simulink model "sfcndemo_csparam"  (Simulink 7.6)
settings: Solver=FixedStepDiscrete  StartTime=0.0  StopTime=Inf  RelTol=1e-3
PostLoadFcn:
  | K1 = 2; K2 = int8(3); MYTYPE = Simulink.AliasType('single');
Description:
  | Context-Sensitive Parameters in C-MEX S-functions
settings Model: Creator=The MathWorks Inc.  CovMetricSettings=d  ExtModeAutoUpdateStatusClock=off  TunableVars=K1,K2  TunableVarsStorageClass=ExportedGlobal,ExportedGlobal  TunableVarsTypeQualifier=,
settings DataIOCC: SaveOutput=off  SaveTime=off  SignalLoggingName=sigsOut
settings OptimizationCC: InlineParams=on  StateBitsets=on  DataBitsets=on  UseTempVars=on  InitFltsAndDblsToZero=on  BufferReusableBoundary=off
settings DebuggingCC: SaveWithParameterizedLinksMsg=none  CheckExecutionContextPreStartOutputMsg=on  CheckExecutionContextRuntimeOutputMsg=on  SolverPrmCheckMsg=none  MultiTaskDSMMsg=warning  MultiTaskCondExecSysMsg=none
settings SFSimCC: SimParseCustomCode=off
settings RTWCC: TLCOptions=-p0  GenerateReport=on  ProcessScript=grt_make_rtw_hook  LaunchReport=on  IncludeERTFirstTime=on
settings CodeAppCC: ForceParamTrailComments=on  CustomSymbolStrFcn=$F$N$M
settings GRTTargetCC: TargetFcnLib=ansi_tfl_tmw.mat

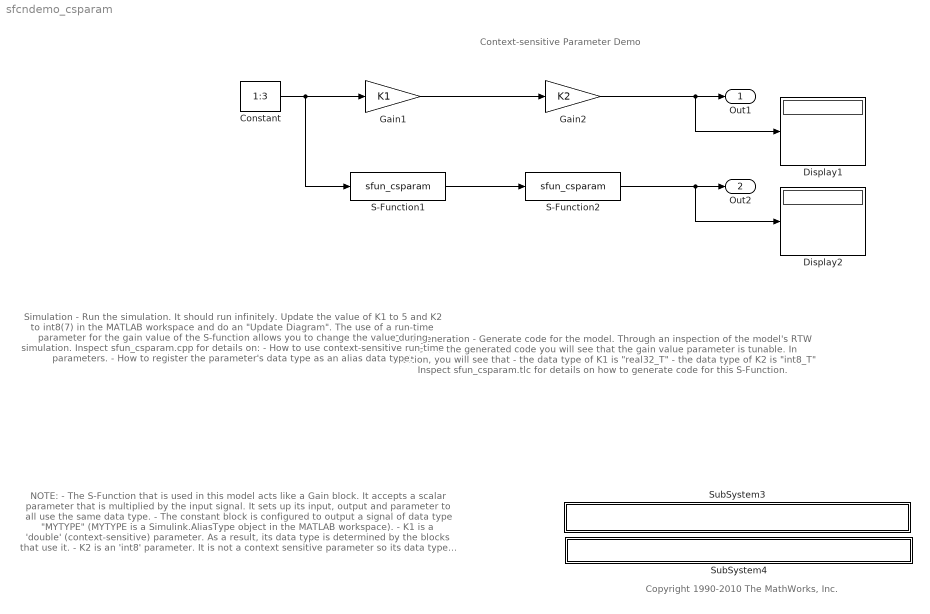
== system sfcndemo_csparam ==
  note: Code generation -
      | Generate code for the model. Through an inspection of the
      | model's RTW file and the generated code you will see that the
      | gain value parameter is tunable.  In addition, you will see that
      | - the data type of K1 is "real32_T"
      | - the data type of K2 is "int8_T"
      |
      | Inspect sfun_csparam.tlc for details on how to generate code
      | for this S-Function.
  note: Simulation -
      | Run the simulation. It should run infinitely.
      | Update the value of K1 to 5 and K2 to int8(7)
      | in the MATLAB workspace and do an "Update Diagram".
      | The use of a run-time parameter for the gain value of the
      | S-function allows you to change the value during simulation.
      |
      | Inspect sfun_csparam.cpp for details on:
      | - How to use context-sensitive run-time parameters.
      | - How to register the parameter's data type as an alias data type.
  note: Context-sensitive Parameter Demo
  note: NOTE:
      | - The S-Function that is used in this model acts like a Gain block.
      |    It accepts a scalar parameter that is multiplied by the input signal.
      |    It sets up its input, output and parameter to all use the same data type.
      | - The constant block is configured to output a signal of data type "MYTYPE"
      |    (MYTYPE is a Simulink.AliasType object in the MATLAB workspace).
      | - K1 is a 'double' (context-sensitive) parameter.
      |    As a result, its data type is determined by the blocks that use it.
      | - K2 is an 'int8' parameter.
      |    It is not a context sensitive parameter so its data type is fixed.
      |    Blocks may need to cast it to the correct data type before using it.
      | - Alias data types are ignored unless you are generating code with 'ert.tlc'.
      |    When using 'ert.tlc', MYTYPE will be preserved in the generated code.
  note: Copyright 1990-2010 The MathWorks, Inc.
  Constant : Constant  Value=1:3  OutDataTypeStr=MYTYPE
  Display1 : Display
  Display2 : Display
  Gain1 : Gain  Gain=K1  SaturateOnIntegerOverflow=on  OutDataTypeStr=Inherit: Same as input  ParamDataTypeStr=Inherit: Same as input
  Gain2 : Gain  Gain=K2  SaturateOnIntegerOverflow=on  OutDataTypeStr=Inherit: Same as input  ParamDataTypeStr=Inherit: Same as input
  S-Function1 : S-Function  FunctionName=sfun_csparam  Parameters=K1  EnableBusSupport=off
  S-Function2 : S-Function  FunctionName=sfun_csparam  Parameters=K2  EnableBusSupport=off
  SubSystem3 : Subsystem  mask{filename=sfun_csparam.cpp}
      mask init:
      | x=sfundemo_maskdisp;
      settings: AttributesFormatString=\n  OpenFcn=sfundemo_openfcn
      mask Display: disp(x);
  SubSystem4 : Subsystem  mask{filename=sfun_csparam.tlc}
      mask init:
      | x=sfundemo_maskdisp;
      settings: AttributesFormatString=\n  OpenFcn=sfundemo_openfcn
      mask Display: disp(x);
  Out1 : Outport
  Out2 : Outport  Port=2
  wires:
  S-Function1/1 -> S-Function2/1
  Constant/1 -> Gain1/1, S-Function1/1
  Gain1/1 -> Gain2/1
  S-Function2/1 -> Out2/1, Display2/1
  Gain2/1 -> Out1/1, Display1/1

== system sfcndemo_csparam/SubSystem3 ==

== system sfcndemo_csparam/SubSystem4 ==
